simulink model "stateflow_commentedOutState"  (R2015b)
settings: Solver=VariableStepAuto  StartTime=0.0  StopTime=10.0  RelTol=1e-3
settings Model: Creator=ladmin  LastModifiedBy=ladmin

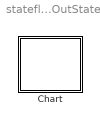
== system stateflow_commentedOutState ==
  Chart : Stateflow chart  TreatAsAtomicUnit=on

== stateflow chart stateflow_commentedOutState/Chart ==
  state ABC
    state DEF
  state GHI [commented out]
  ABC -> GHI [commented out] : [Label 2]
  (default) -> ABC [order 2]
  (default) -> (junction 4) [order 1]
  GHI -> ABC [commented out] : MyLabel
